simulink model "lab8"  (R2017b)
settings: Solver=ode4  StartTime=0.0  StopTime=100  FixedStep=0.0001  RelTol=1e-3
undefined symbols (not defined in the file or in its folder): i, k, x
settings Model: Creator=ayushi  LastModifiedBy=ayushi

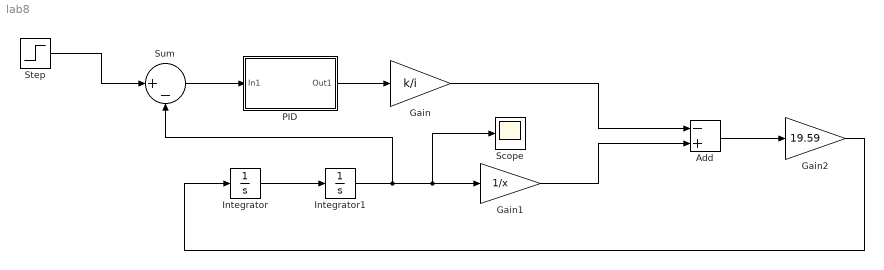
== system lab8 ==
  Add : Sum  Inputs=-+
  Gain : Gain  Gain=k/i
  Gain1 : Gain  Gain=1/x
  Gain2 : Gain  Gain=19.59
  Integrator : Integrator
  Integrator1 : Integrator
  "PID " : Subsystem
  Scope : Scope
  Step : Step  After=0.009  SampleTime=0
  Sum : Sum  Inputs=|+-
  wires:
  Step/1 -> Sum/1
  Gain/1 -> Add/1
  Integrator/1 -> Integrator1/1
  Integrator1/1 -> Sum/2, Scope/1, Gain1/1
  Gain1/1 -> Add/2
  Add/1 -> Gain2/1
  Gain2/1 -> Integrator/1
  Sum/1 -> "PID "/1(In1)
  "PID "/1(Out1) -> Gain/1

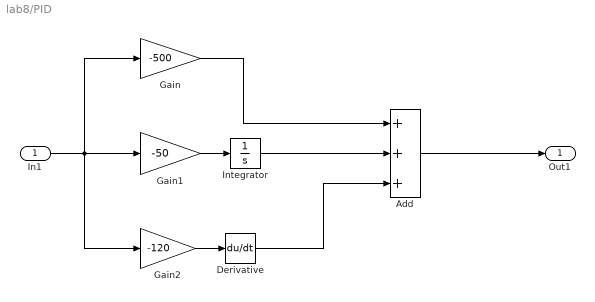
== system lab8/PID  ==
  In1 : Inport
  Add : Sum  Inputs=+++
  Derivative : Derivative
  Gain : Gain  Gain=-500
  Gain1 : Gain  Gain=-50
  Gain2 : Gain  Gain=-120
  Integrator : Integrator
  Out1 : Outport
  wires:
  Gain/1 -> Add/1
  Gain2/1 -> Derivative/1
  Derivative/1 -> Add/3
  Integrator/1 -> Add/2
  Add/1 -> Out1/1
  In1/1 -> Gain2/1, Gain1/1, Gain/1
  Gain1/1 -> Integrator/1
